simulink model "Exercise1"  (R2025a)
settings: Solver=VariableStepAuto  StartTime=0.0  StopTime=0.5  RelTol=1e-3
undefined symbols (not defined in the file or in its folder): dspblkCoreblockFVToolHelper, gcbh
libraries: dspfdesign x3, dspsrcs4 x2, dspsigops x1, spspowerguiLib x1
settings Model: Creator=francoisdesautels  LastModifiedBy=francoisdesautels

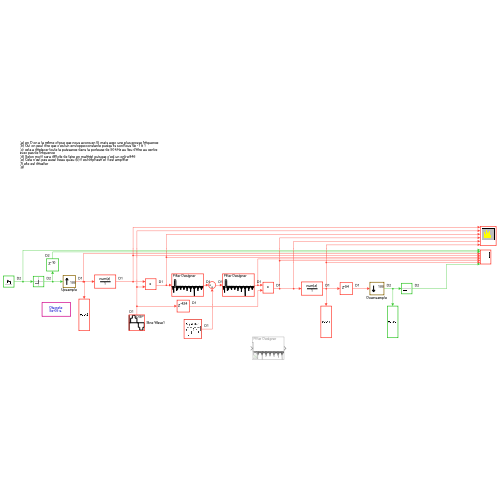
[thumbnail: Simulink's stored preview of the top-level diagram]
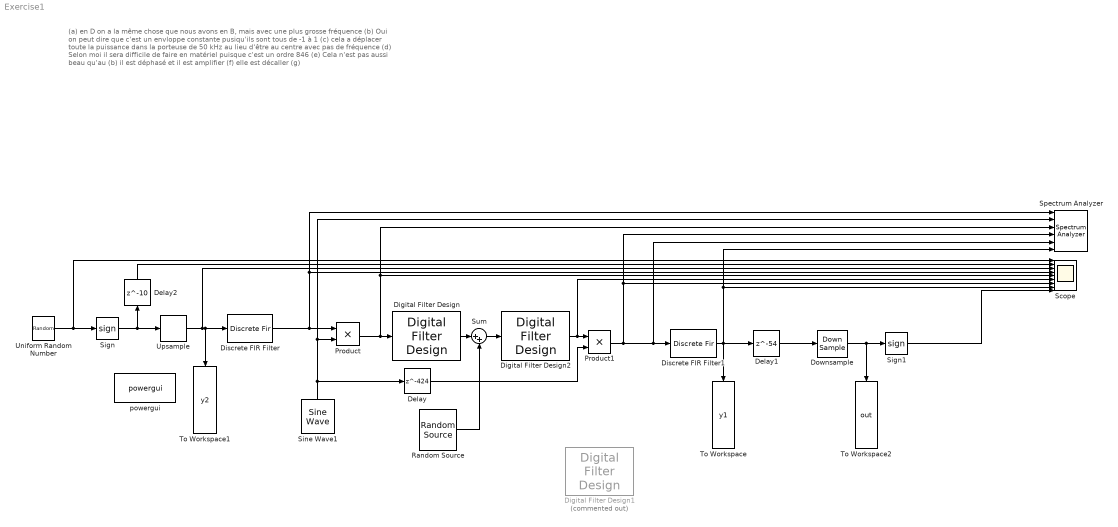
== system Exercise1 ==
  note: (a) en D on a la même chose que nous avons en B, mais avec une plus grosse fréquence
      | (b) Oui on peut dire que c'est un envloppe constante pusiqu'ils sont tous de -1 à 1
      | (c) cela a déplacer toute la puissance dans la porteuse de 50 kHz au lieu d'être au centre avec pas de fréquence
      | (d) Selon moi il sera difficile de faire en matériel puisque c'est un ordre 846
      | (e) Cela n'est pas aussi beau qu'au (b) il est déphasé et il est amplifier
      | (f) elle est décaller
      | (g)
  Delay : Delay  DelayLength=424
  Delay1 : Delay  DelayLength=54
  Delay2 : Delay  DelayLength=10
  Digital Filter Design : dspfdesign/Digital Filter Design  mwdsp_browser_bugfix_var=off
  Digital Filter Design1 : dspfdesign/Digital Filter Design  Commented=on  mwdsp_browser_bugfix_var=off
  Digital Filter Design2 : dspfdesign/Digital Filter Design  mwdsp_browser_bugfix_var=off
  Discrete FIR Filter : DiscreteFir  LoadFcn=dspblkCoreblockFVToolHelper(gcbh,'load');  Coefficients=ones(1,100)
      settings: CopyFcn=dspblkCoreblockFVToolHelper(gcbh,'copy');  DeleteFcn=dspblkCoreblockFVToolHelper(gcbh,'close');  ModelCloseFcn=dspblkCoreblockFVToolHelper(gcbh,'close');  PreSaveFcn=dspblkCoreblockFVToolHelper(gcbh,'presave');  PostSaveFcn=dspblkCoreblockFVToolHelper(gcbh,'postsave');  CloseFcn=dspblkCoreblockFVToolHelper(gcbh,'close');
  Discrete FIR Filter1 : DiscreteFir  LoadFcn=dspblkCoreblockFVToolHelper(gcbh,'load');  Coefficients=ones(1,100)
      settings: CopyFcn=dspblkCoreblockFVToolHelper(gcbh,'copy');  DeleteFcn=dspblkCoreblockFVToolHelper(gcbh,'close');  ModelCloseFcn=dspblkCoreblockFVToolHelper(gcbh,'close');  PreSaveFcn=dspblkCoreblockFVToolHelper(gcbh,'presave');  PostSaveFcn=dspblkCoreblockFVToolHelper(gcbh,'postsave');  CloseFcn=dspblkCoreblockFVToolHelper(gcbh,'close');
  Downsample : DownSample  N=100  RateOptions=Allow multirate processing
  Product : Product
  Product1 : Product
  Random Source : dspsrcs4/Random Source  SrcType=Gaussian  MinVal=0  MaxVal=1  MeanVal=0  VarVal=1  RepMode=Specify seed  rawSeed=1  IsInherit=off  SampTime=1/1000000  SampFrame=1  OutComplex=Real  DataType=double  SimulateUsing=Interpreted execution
  Scope : Scope  NumInputPorts=9
      settings: ActiveDisplayYMinimum=-1.1698560364941972  ActiveDisplayYMaximum=1.6010341967824271
  Sign : Signum
  Sign1 : Signum
  Sine Wave1 : dspsrcs4/Sine Wave  Amplitude=1  Frequency=50000  Phase=pi/2  SampleMode=Discrete  OutComplex=Real  CompMethod=Trigonometric fcn  TableSize=Speed  SampleTime=1/1000000  SamplesPerFrame=1  ResetState=Restart at time zero  OutputFrames=off  dataType=double  wordLen=16  udDataType=sfix(16)  fracBitsMode=Best precision  numFracBits=15  OutDataTypeStr=double  LastOutDataTypeStr=double
  Spectrum Analyzer : SpectrumAnalyzer  NumInputPorts=6  WindowPosition=[1109.000000,602.000000,979.000000,638.000000,]  Visible=on  ScopeFrameLocation=window  SpectrumType=Power density  WindowInvariantSamplesPerUpdate=on  Span=1000000  StartFrequency=-500000  StopFrequency=500000  SpectrumUnits=dBm/Hz  MaximizeAxes=Off  YLimits=[-295.7819 49.2638]  ShowLegend=on
  Sum : Sum  Inputs=|++
  To Workspace : ToWorkspace  VariableName=y1  SampleTime=-1
      settings: Save2DSignal=2-D array (concatenate along first dimension)
  To Workspace1 : ToWorkspace  VariableName=y2  SampleTime=-1
      settings: Save2DSignal=2-D array (concatenate along first dimension)
  To Workspace2 : ToWorkspace  VariableName=out  SampleTime=-1
      settings: Save2DSignal=2-D array (concatenate along first dimension)
  Uniform Random Number : UniformRandomNumber  SampleTime=1/10000
  Upsample : dspsigops/Upsample  FactorSource=Dialog parameter  N=100  Nmax=16  phase=0  RateOptions=Allow multirate processing  ic=0  mode=Unused parameter value
      settings: LibrarySourceBlock=dsphdlsupportsigops/Upsample
  powergui : spspowerguiLib/powergui  Priority=1  SimulationMode=Discrete  SampleTime=50e-6  frequency=60  Iterations=50  frequencyindice=60  Pbase=100e6  ErrMax=1e-4  UnitsV=kV  UnitsW=MW  buscounter=0  FunctionMessages=off  echomessages=off  EnableUseOfTLC=off  CurrentSourceSwitches=off  DisableSnubberDevices=off  DisableRonSwitches=off  DisableVfSwitches=off  DisplayEquations=off  AutomaticDiscreteSolvers=off  SolverType=Tustin/Backward Euler (TBE)  Interpol=off  ExternalGateDelay=off  methode=off  Ts=100  x0status=blocks  SPID=on  SwTol=0  HookPort=off  NonlinearTolerance=1e-4  nMaxIteration=100  ContinueOnMaxIteration=off  RestoreLinks=warning  ResistiveCurrentMeasurement=off  Frange=[0:2:500]  Ylog=off  Xlog=on  ShowGrid=off  save=off  variable=ZData  structure=0  ZoomFFT=off  StartTime=0.0  cycles=1  DisplayStyle=1  fundamental=60  FreqAxis=off  MaxFrequency=1000  frequencyindicesteady=1  RmsSteady=1  display=off
  wires:
  Upsample/1 -> To Workspace1/1, Discrete FIR Filter/1, Scope/3
  Sign/1 -> Upsample/1, Delay2/1
  Uniform Random Number/1 -> Scope/1, Sign/1
  Product/1 -> Spectrum Analyzer/3, Scope/5, Digital Filter Design/1
  Sine Wave1/1 -> Spectrum Analyzer/2, Product/2, Delay/1
  Delay/1 -> Product1/2
  Product1/1 -> Spectrum Analyzer/5, Discrete FIR Filter1/1, Spectrum Analyzer/4, Scope/7
  Discrete FIR Filter1/1 -> Delay1/1, To Workspace/1, Spectrum Analyzer/6, Scope/8
  Delay1/1 -> Downsample/1
  Downsample/1 -> To Workspace2/1, Sign1/1
  Sign1/1 -> Scope/9
  Delay2/1 -> Scope/2
  Discrete FIR Filter/1 -> Spectrum Analyzer/1, Scope/4, Product/1
  Random Source/1 -> Sum/2
  Digital Filter Design2/1 -> Scope/6, Product1/1
  Digital Filter Design/1 -> Sum/1
  Sum/1 -> Digital Filter Design2/1
